simulink model "model02_2013a"  (Simulink 8.1)
settings: Solver=FixedStepDiscrete  StartTime=0.0  StopTime=10.0  FixedStep=0.1  RelTol=1e-3
undefined symbols (not defined in the file): sigbuilder_block
settings Model: Creator=ladmin  LastModifiedBy=ladmin
settings OptimizationCC: ExpressionDepthLimit=128  InitFltsAndDblsToZero=on
settings DebuggingCC: SaveWithParameterizedLinksMsg=none  SignalResolutionControl=TryResolveAllWithWarning  MultiTaskDSMMsg=warning  MultiTaskCondExecSysMsg=none  StateNameClashWarn=none  StrictBusMsg=Warning
settings RTWCC: IncludeERTFirstTime=on
settings GRTTargetCC: TargetFcnLib=ansi_tfl_tmw.mat

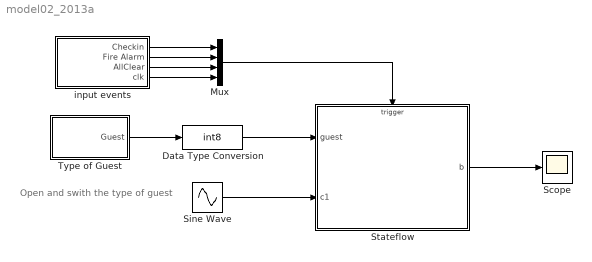
== system model02_2013a ==
  note: Open and swith the
      | type of guest
  Data Type Conversion : DataTypeConversion  OutDataTypeStr=int8
  Mux : Mux
  Scope : Scope
      settings: TimeRange=10  YMin=-4  YMax=4
  Sine Wave : Sin  Amplitude=2  Frequency=10  Samples=20  SampleTime=0.1
  Stateflow : Stateflow chart  TreatAsAtomicUnit=on
      settings: PermitHierarchicalResolution=ParametersOnly
  Type of Guest : Subsystem  Tag=STV Subsys  LoadFcn=sigbuilder_block('load');  StartFcn=sigbuilder_block('start');  StopFcn=sigbuilder_block('stop');  ClipboardFcn=sigbuilder_block('clipboard');  mask(Sigbuilder block){}
      mask help: Sigbuilder GUI
      mask init:
      | if ~strcmp(get_param(bdroot(gcbh),'SimulationStatus'),'stopped') tuvar = sigbuilder_block('maskInit'); end
      settings: CopyFcn=sigbuilder_block('copy');  DeleteFcn=sigbuilder_block('delete');  ModelCloseFcn=sigbuilder_block('modelClose');  PreSaveFcn=sigbuilder_block('preSave');  PauseFcn=sigbuilder_block('pause')  ContinueFcn=sigbuilder_block('continue')  NameChangeFcn=sigbuilder_block('namechange');  OpenFcn=sigbuilder_block('open',[147.75 115.5 550.5 360 ]);  CloseFcn=sigbuilder_block('close');
      mask Display: plot(0,0,100,100,[10,10,40,40,10],[80,20,20,80,80],[40,10],[50,50], [40,27,10],[65,72,56],[40,25,25,10],[28,28,43,43]);
  input events : Subsystem  Tag=STV Subsys  LoadFcn=sigbuilder_block('load');  StartFcn=sigbuilder_block('start');  StopFcn=sigbuilder_block('stop');  ClipboardFcn=sigbuilder_block('clipboard');  mask(Sigbuilder block){}
      mask help: Sigbuilder GUI
      mask init:
      | if ~strcmp(get_param(bdroot(gcbh),'SimulationStatus'),'stopped') tuvar = sigbuilder_block('maskInit'); end
      settings: CopyFcn=sigbuilder_block('copy');  DeleteFcn=sigbuilder_block('delete');  ModelCloseFcn=sigbuilder_block('modelClose');  PreSaveFcn=sigbuilder_block('preSave');  PauseFcn=sigbuilder_block('pause')  ContinueFcn=sigbuilder_block('continue')  NameChangeFcn=sigbuilder_block('namechange');  OpenFcn=sigbuilder_block('open',[121.5 125.25 549.75 360 ]);  CloseFcn=sigbuilder_block('close');
      mask Display: plot(0,0,100,100,[10,10,40,40,10],[80,20,20,80,80],[40,10],[50,50], [40,27,10],[65,72,56],[40,25,25,10],[28,28,43,43]);
  wires:
  Type of Guest/1(Guest) -> Data Type Conversion/1
  Sine Wave/1 -> Stateflow/2(c1)
  Mux/1 -> Stateflow/Trigger
  input events/1(Checkin) -> Mux/1
  input events/2(Fire Alarm) -> Mux/2
  input events/3(AllClear) -> Mux/3
  Data Type Conversion/1 -> Stateflow/1(guest)
  Stateflow/1(b) -> Scope/1
  input events/4(clk) -> Mux/4

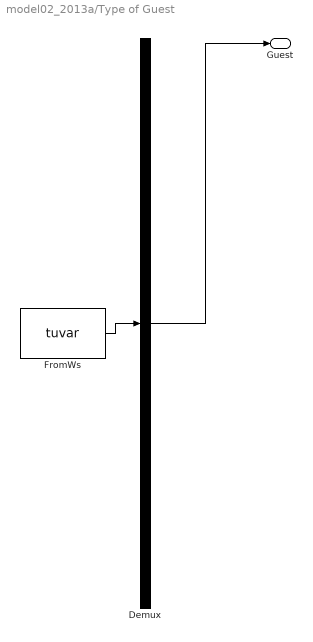
== system model02_2013a/Type of Guest ==
  Demux : Demux  Tag=STV Demux  Outputs=1
  FromWs : FromWorkspace  Tag=STV FromWs  VariableName=tuvar  SampleTime=0  SigBuilderData=DataTag0  VnvData=DataTag1
      SigBuilderData=|
      | common.afterFinalStr = 'Extrapolate'
      | common.sampleTime = 0
      | dataSet(1).timeRange = [0 10]
      | dataSet(1).name = 'Nonsmoking'
      | dataSet(2).timeRange = [0 10]
      | dataSet(2).name = 'Smoking'
      | dataSet(3).timeRange = [0 10]
      | dataSet(3).name = 'Rich'
      | dataSet(4).timeRange = [0 10]
      | dataSet(4).name = 'Family'
      | sbobj.Groups(1).Name = 'Nonsmoking'
      | sbobj.Groups(1).Signals.Name = 'Guest'
      | sbobj.Groups(1).Signals.XData = [0 10]
      | sbobj.Groups(1).Signals.YData = [0 0]
      | sbobj.Groups(2).Name = 'Smoking'
      | sbobj.Groups(2).Signals.Name = 'Guest'
      | sbobj.Groups(2).Signals.XData = [0 10]
      | sbobj.Groups(2).Signals.YData = [1 1]
      | sbobj.Groups(3).Name = 'Rich'
      | sbobj.Groups(3).Signals.Name = 'Guest'
      | sbobj.Groups(3).Signals.XData = [0 10]
      | sbobj.Groups(3).Signals.YData = [2 2]
      | sbobj.Groups(4).Name = 'Family'
      | sbobj.Groups(4).Signals.Name = 'Guest'
      | sbobj.Groups(4).Signals.XData = [0 10]
      | sbobj.Groups(4).Signals.YData = [3 3]
  Guest : Outport  Tag=STV Outport
  wires:
  Demux/1 -> Guest/1
  FromWs/1 -> Demux/1

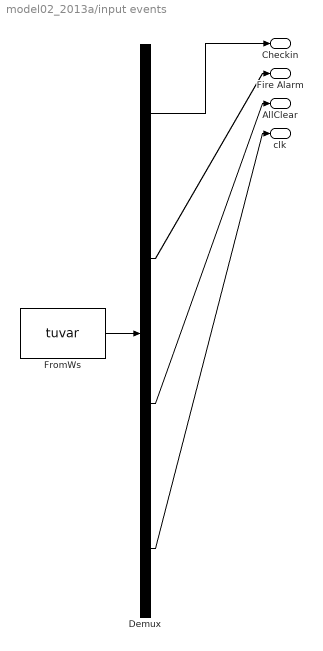
== system model02_2013a/input events ==
  Demux : Demux  Tag=STV Demux
  FromWs : FromWorkspace  Tag=STV FromWs  VariableName=tuvar  SampleTime=0  SigBuilderData=DataTag2  VnvData=DataTag3
      SigBuilderData=|
      | common.afterFinalStr = 'Extrapolate'
      | common.sampleTime = 0
      | dataSet.timeRange = [0 10]
      | dataSet.name = 'Group 1'
      | sbobj.Groups.Name = 'Group 1'
      | sbobj.Groups.Signals(1).Name = 'Checkin'
      | sbobj.Groups.Signals(1).XData = [0 1 1 10]
      | sbobj.Groups.Signals(1).YData = [0 0 1 1]
      | sbobj.Groups.Signals(2).Name = 'Fire Alarm'
      | sbobj.Groups.Signals(2).XData = [0 5 5 6 6 10]
      | sbobj.Groups.Signals(2).YData = [0 0 1 1 0.02 0.02]
      | sbobj.Groups.Signals(3).Name = 'AllClear'
      | sbobj.Groups.Signals(3).XData = [0 8 8 10]
      | sbobj.Groups.Signals(3).YData = [0 0 1 1]
      | sbobj.Groups.Signals(4).Name = 'clk'
      | sbobj.Groups.Signals(4).XData = [0 0.25 0.25 0.5 0.5 0.75 0.75 1 1 1.25 1.25 1.5 1.5 1.75 1.75 2 2 2.25 2.25 2.5 2.5 2.75 2.75 3 3 3.25 3.25 3.5 3.5 3.75 3.75 4 4 4.25 4.25 4.5 4.5 4.75 4.75 5 5 5.25 5.25 5.5 5.5 5.75 5.75 6 6 6.25 6.25 6.5 6.5 6.75 6.75 7 7 7.25 7.25 7.5 7.5 7.75 7.75 8 8 8.25 8.25 8.5 8.5 8.75 8.75 9 9 9.25 9.25 9.5 9.5 9.75 9.75 10]
      | sbobj.Groups.Signals(4).YData = [1 1 0 0 1 1 0 0 0 0 0 0 1 1 0 0 1 1 0 0 1 1 0 0 1 1 0 0 1 1 0 0 1 1 0 0 1 1 0 0 0 0 0 0 1 1 0 0 1 1 0 0 1 1 0 0 1 1 0 0 1 1 0 0 0 0 0 0 1 1 0 0 1 1 0 0 1 1 0 0]
  Checkin : Outport  Tag=STV Outport
  Fire Alarm : Outport  Tag=STV Outport  Port=2
  AllClear : Outport  Tag=STV Outport  Port=3
  clk : Outport  Tag=STV Outport  Port=4
  wires:
  Demux/1 -> Checkin/1
  FromWs/1 -> Demux/1
  Demux/2 -> Fire Alarm/1
  Demux/3 -> AllClear/1
  Demux/4 -> clk/1

== stateflow chart Stateflow ==
  state HotelStateflow
    (history)
    state NonSmokingRoom
      entry: b=unpack();
      during: b=callhome();
      exit: b=pack();
    state SmokingRoom
    state ExecutiveSuite
      state MasterBed
      state SecondBed
      (default) -> HotelStateflow.ExecutiveSuite.MasterBed
      HotelStateflow.ExecutiveSuite.SecondBed -> HotelStateflow.ExecutiveSuite.MasterBed : [c1]
      HotelStateflow.ExecutiveSuite.MasterBed -> HotelStateflow.ExecutiveSuite.SecondBed : [c1]
    state FamilySuite
      state MasterBed [parallel]
        settings: executionOrder=1
      state SecondBed [parallel]
        settings: executionOrder=2
    state y=is_family(x) [function]
      (default) -> (junction 35)
      (junction 35) -> (junction 36) [order 1] : [x>2]
      (junction 35) -> (junction 37) [order 2] : {y=0;}
      (junction 36) -> (junction 38) : {y=1;}
    state y=pack [function]
      (default) -> (junction 45)
      (junction 45) -> (junction 46) : {
          | /* Condition #1 */
          | aVarTruthTableCondition_1 = (c1>1);
          | }
      (junction 46) -> (junction 47) [order 1] : [aVarTruthTableCondition_1]   /* D1 */
      (junction 47) -> (junction 48) : {
          | /* Action 1 */
          | y=2;
          | }
      (junction 46) -> (junction 49) [order 2]
      (junction 49) -> (junction 50) [order 1] : [!aVarTruthTableCondition_1]   /* D2 */
      (junction 50) -> (junction 51) : {
          | /* Action 2 */
          | y=1;
          | }
      (junction 49) -> (junction 52) [order 2]
    state y=unpack [function]
      (default) -> (junction 63)
      (junction 63) -> (junction 64) [order 1] : [c1<0]
      (junction 64) -> (junction 65) : {y=3;}
      (junction 63) -> (junction 66) [order 2] : {y=4;}
    state wait
    (junction 24) -> NonSmokingRoom [order 2]
    (default) -> wait
    wait -> (junction 22) : checkin
    (junction 22) -> (junction 23) [order 2]
    (junction 23) -> (junction 24) [order 2]
    (junction 22) -> FamilySuite [order 1] : [is_family(guest)]
    (junction 23) -> ExecutiveSuite [order 1] : [guest==rich]
    (junction 24) -> SmokingRoom [order 1] : [guest==smoking]
  state AssemblyPoint
  (default) -> HotelStateflow
  HotelStateflow -> AssemblyPoint : Firealarm
  AssemblyPoint -> HotelStateflow : Allclear
  data: x function_input double; y function_output double; y function_output double; aVarTruthTableCondition_1 temporary boolean =0; y function_output double; y function_output double; guest input double; rich local int8 =2; smoking local int8 =1; c1 input double; b output double
  events: E local RISING_EDGE_EVENT; checkin input RISING_EDGE_EVENT; Firealarm input RISING_EDGE_EVENT; Allclear input RISING_EDGE_EVENT; clk input RISING_EDGE_EVENT
  function y=callhome:
    | function y=callhome()
    | 
    | %do some calculations
    |  
    | y=c1*2;
